simulink library "SinglePhase_Load"  (Simulink 7.8)
settings: Solver=ode45  StartTime=0.0  StopTime=10.0  RelTol=1e-3
libraries: powerlib x3, powerlib_extras x1
settings Model: Creator=MA25949  LastModifiedBy=MA25949

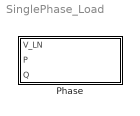
== system SinglePhase_Load ==
  "Phase " : Subsystem

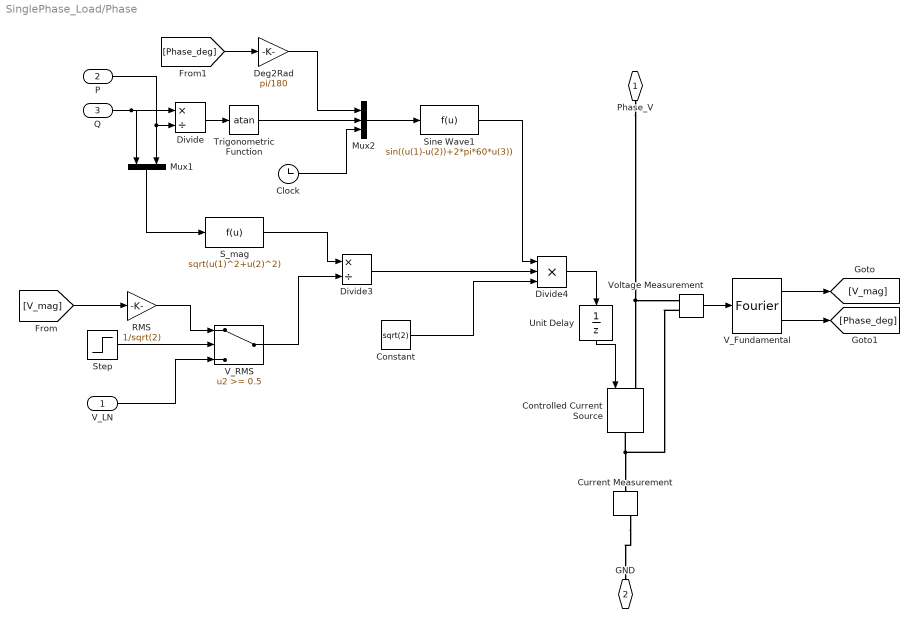
== system SinglePhase_Load/Phase  ==
  V_LN : Inport
  P : Inport  Port=2
  Q : Inport  Port=3
  Clock : Clock
      settings: Decimation=100000
  Constant : Constant  Value=sqrt(2)
  Controlled Current Source : powerlib/Electrical Sources/Controlled Current Source  Initialize=on  Source_Type=AC  Amplitude=0  Phase=0  Frequency=0  Measurements=None
  Current Measurement : powerlib/Measurements/Current Measurement  PhasorSimulation=off  OutputType=Complex  PSBequivalent=0
  Deg2Rad : Gain  Gain=pi/180
  Divide : Product  Inputs=*/
  Divide3 : Product  Inputs=*/
  Divide4 : Product  Inputs=***
  Mux1 : Mux  Inputs=2
  Mux2 : Mux  Inputs=3
  RMS : Gain  Gain=1/sqrt(2)
  S_mag : Fcn  Expr=sqrt(u(1)^2+u(2)^2)
  Sine Wave1 : Fcn  Expr=sin((u(1)-u(2))+2*pi*60*u(3))
  Step : Step  Time=0.02  SampleTime=0
  Trigonometric Function : Trigonometry  Operator=atan
  Unit Delay : UnitDelay  SampleTime=-1
  V_Fundamental : powerlib_extras/Measurements/Fourier  f1=60  n=1
  V_RMS : Switch  Threshold=0.5
  Voltage Measurement : powerlib/Measurements/Voltage Measurement  PhasorSimulation=off  OutputType=Complex  PSBequivalent=0
  Phase_V : PMIOPort  Port=1  Side=Right
  GND : PMIOPort  Port=2  Side=Right
  wires:
  Q/1 -> Divide/1, Mux1/1
  P/1 -> Divide/2, Mux1/2
  Divide/1 -> Trigonometric Function/1
  Trigonometric Function/1 -> Mux2/2
  Mux1/1 -> S_mag/1
  S_mag/1 -> Divide3/1
  Constant/1 -> Divide4/3
  Divide4/1 -> Unit Delay/1
  Unit Delay/1 -> Controlled Current Source/1
  Voltage Measurement/1 -> V_Fundamental/1
  Mux2/1 -> Sine Wave1/1
  Sine Wave1/1 -> Divide4/1
  Step/1 -> V_RMS/2
  V_LN/1 -> V_RMS/3
  Clock/1 -> Mux2/3
  V_RMS/1 -> Divide3/2
  Divide3/1 -> Divide4/2
  V_Fundamental/1 -> [V_mag]
  [V_mag] -> RMS/1
  RMS/1 -> V_RMS/1
  V_Fundamental/2 -> [Phase_deg]
  [Phase_deg] -> Deg2Rad/1
  Deg2Rad/1 -> Mux2/1
  connections:
  Phase_V/RConn1 -- Controlled Current Source/LConn1 -- Voltage Measurement/LConn1
  Voltage Measurement/LConn2 -- Controlled Current Source/RConn1 -- Current Measurement/LConn1
  Current Measurement/RConn1 -- GND/RConn1
